simulink model "Super1"  (Simulink 5.0)
settings: Solver=ode45  StartTime=0.0  StopTime=10.0  RelTol=1e-3
settings Model: Creator=scaife  LastModifiedBy=scaife  ExtModeAutoUpdateStatusClock=off

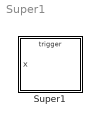
== system Super1 ==
  Super1 : Stateflow chart

== stateflow chart Super1 ==
  state A
  state B
  state C
    state C1
    state C2
    C1 -> C2 : F
    C2 -> C1 : F
    (default) -> C1
  state D
  (default) -> A
  A -> (junction 10) : E
  C2 -> (junction 9) : E[x<2]
  C1 -> B : E
  B -> C2 : E
  (junction 9) -> D : [x<>0]
  (junction 9) -> A : [x==0]
  D -> A : F
  (junction 10) -> C1 : [x==0]
  (junction 10) -> D : [x<>0]
  data: x input int32
  events: E input EITHER_EDGE_EVENT; F input EITHER_EDGE_EVENT
